simulink model "BMS_test_SOC_multi_cell"  (R2024a)
settings: Solver=FixedStepAuto  StartTime=0.0  StopTime=BMS_time1(end)  FixedStep=.1  RelTol=1e-3
settings Model: DataDictionary=SOXDictionary.sldd  PacingRate=100  Creator=mmackenzie  LastModifiedBy=mmackenzie
settings OptimizationCC: DefaultUnderspecifiedDataType=single
settings DebuggingCC: ParamPrecisionLossAbsoluteDiffThreshold=1e-10  ParamPrecisionLossRelativeDiffThreshold=1e-6  AllowSymbolicDim=off

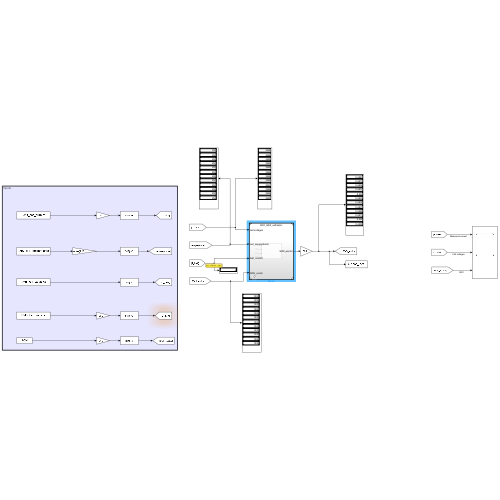
[thumbnail: Simulink's stored preview of the top-level diagram]
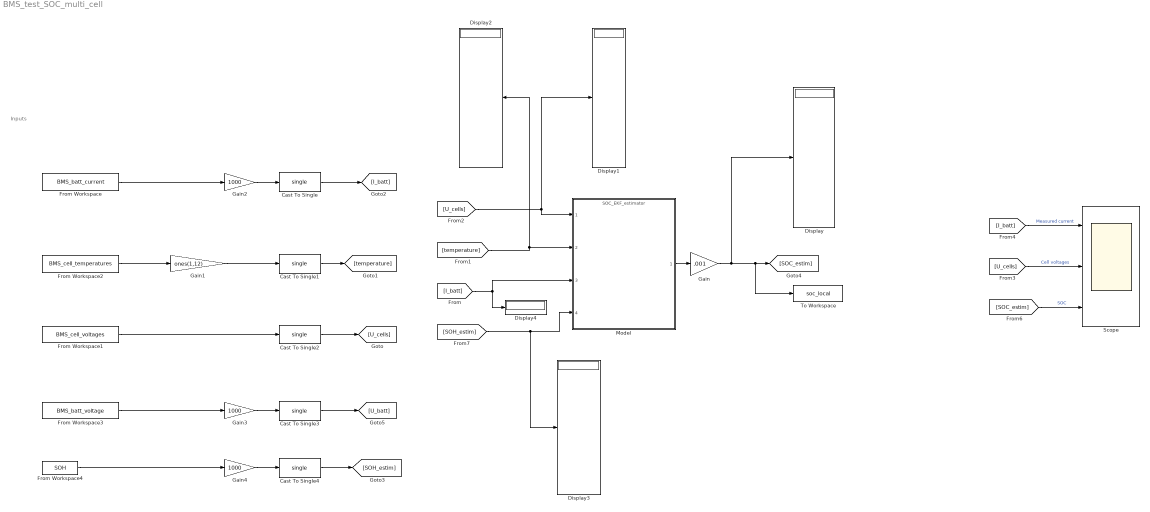
== system BMS_test_SOC_multi_cell ==
  note: Inputs
  Cast To Single{,1..4} (5 alike) : DataTypeConversion  OutDataTypeStr=single  SaturateOnIntegerOverflow=off  RndMeth=Floor
  Display{,1..4} (5 alike) : Display
  From Workspace : FromWorkspace  VariableName=BMS_batt_current  SampleTime=.1
  From Workspace1 : FromWorkspace  VariableName=BMS_cell_voltages  SampleTime=.1
  From Workspace2 : FromWorkspace  VariableName=BMS_cell_temperatures  SampleTime=.1
  From Workspace3 : FromWorkspace  VariableName=BMS_batt_voltage  SampleTime=.1
  From Workspace4 : FromWorkspace  VariableName=SOH  SampleTime=.1
  Gain : Gain  Gain=.001
  Gain1 : Gain  Gain=ones(1,12)
  Gain2 : Gain  Gain=1000
  Gain3 : Gain  Gain=1000
  Gain4 : Gain  Gain=1000
  Model : ModelReference  ModelNameDialog=SOC_EKF_estimator.slx  SimulationMode=Normal  ModelReferenceVersion=1.36
  Scope : Scope  NumInputPorts=3
  To Workspace : ToWorkspace  VariableName=soc_local  SaveFormat=Timeseries  SampleTime=-1
  wires:
  [I_batt] -> Scope/1  "Measured current"
  Model/1 -> Gain/1
  [SOC_estim] -> Scope/3  "SOC"
  From Workspace4/1 -> Gain4/1
  [I_batt] -> Model/3, Display4/1
  Gain/1 -> To Workspace/1, [SOC_estim], Display/1
  From Workspace/1 -> Gain2/1
  From Workspace1/1 -> Cast To Single2/1
  Gain3/1 -> Cast To Single3/1
  Gain4/1 -> Cast To Single4/1
  Cast To Single/1 -> [I_batt]
  Cast To Single1/1 -> [temperature]
  Cast To Single2/1 -> [U_cells]
  Cast To Single3/1 -> [U_batt]
  Cast To Single4/1 -> [SOH_estim]
  [U_cells] -> Scope/2  "Cell voltages"
  From Workspace3/1 -> Gain3/1
  From Workspace2/1 -> Gain1/1
  Gain1/1 -> Cast To Single1/1
  [U_cells] -> Model/1, Display1/1
  [temperature] -> Model/2, Display2/1
  [SOH_estim] -> Model/4, Display3/1
  Gain2/1 -> Cast To Single/1
